simulink model "Powertrain_model_HEV_21a"  (R2021a)
settings: Solver=VariableStepAuto  StartTime=0.0  StopTime=tspan  RelTol=1e-3
values from neighbouring files (symbols this model uses):
  bsfc_idle_CE = 31.7e03    (= 31700)    [Sim_script.m]
  bsfc_idle_GE = 4.96e03    (= 4960)    [Sim_script.m]
  DR = 5.213    [Sim_script.m]
  drawn_pow_M = 464.6018    [Sim_script.m]
  Gensetdata = Gensetdata1    [Sim_script.m]
  motor_eff = motor_eff_PMSM    [Sim_script.m]
  Trans_In = 24.086    [Sim_script.m]
  tspan = 10800    [Sim_script.m]
  w_CE_idle = 400    [Sim_script.m]
undefined symbols (not defined in the file or in its folder): dailyloadl, eta_EM_map, MaxLimit, resT_hybrid_bollard, resT_hybrid_free, resT_hybrid_tow, T_EM_col, T_EM_max, w_EM_row
libraries: pid_lib x1
settings Model: Creator=user  LastModifiedBy=olsonsao
settings SolverCC: AlgebraicLoopSolver=TrustRegion

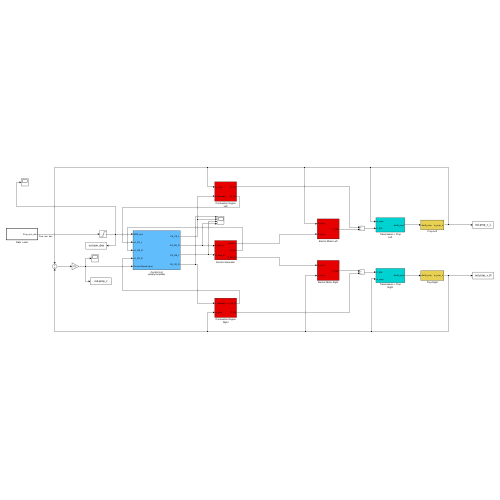
[thumbnail: Simulink's stored preview of the top-level diagram]
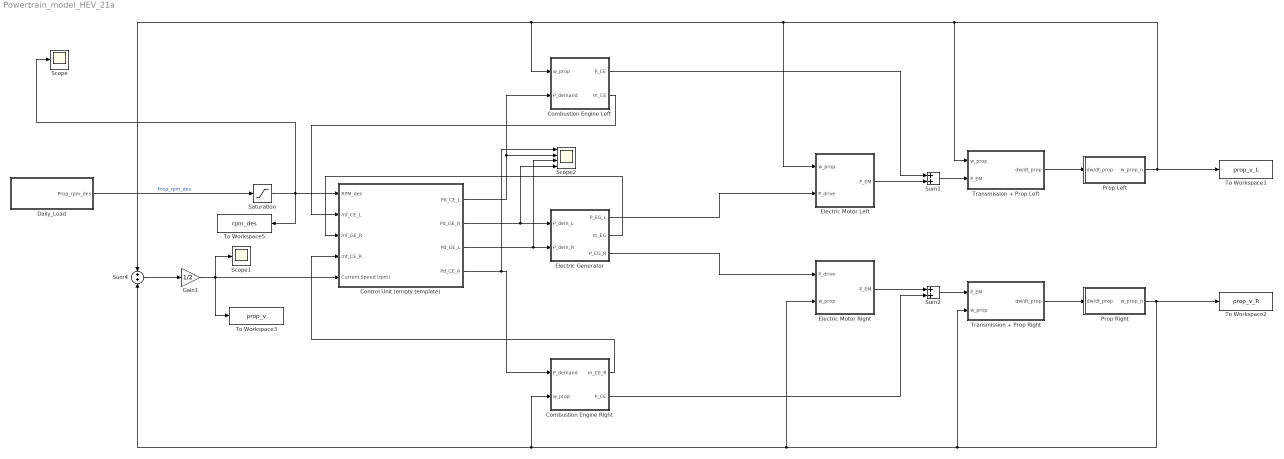
== system Powertrain_model_HEV_21a ==
  Combustion Engine Left : Subsystem  Tag=combustion engine
  Combustion Engine Right : Subsystem  Tag=combustion engine
  Control Unit (empty template) : Subsystem  Tag=control unit
  Daily_Load : Subsystem  TreatAsAtomicUnit=on
  "Electric Generator " : Subsystem
  Electric Motor Left : Subsystem
  Electric Motor Right : Subsystem
  Gain1 : Gain  Gain=1/2
  Prop Left : Subsystem
  Prop Right : Subsystem
  Saturation : Saturate  UpperLimit=inf  LowerLimit=w_CE_idle/DR
  Scope : Scope
  Scope1 : Scope
  Scope2 : Scope  NumInputPorts=4
  Sum1 : Sum
  Sum2 : Sum
  Sum4 : Sum  Inputs=+|+
  To Workspace1 : ToWorkspace  VariableName=prop_v_L  SampleTime=-1
      settings: Save2DSignal=2-D array (concatenate along first dimension)
  To Workspace2 : ToWorkspace  VariableName=prop_v_R  SampleTime=-1
      settings: Save2DSignal=2-D array (concatenate along first dimension)
  To Workspace3 : ToWorkspace  VariableName=prop_v  SampleTime=-1
      settings: Save2DSignal=2-D array (concatenate along first dimension)
  To Workspace5 : ToWorkspace  VariableName=rpm_des  SampleTime=-1
      settings: Save2DSignal=2-D array (concatenate along first dimension)
  Transmission + Prop Left : Subsystem
  Transmission + Prop Right : Subsystem
  wires:
  Transmission + Prop Left/1(dw/dt_prop) -> Prop Left/1(dw/dt_prop)
  Transmission + Prop Right/1(dw/dt_prop) -> Prop Right/1(dw/dt_prop)
  Prop Left/1(w_prop_n) -> Transmission + Prop Left/1(w_prop), Electric Motor Left/1(w_prop), Sum4/1, Combustion Engine Left/1(w_prop), To Workspace1/1
  Electric Motor Right/1(P_EM) -> Sum2/1
  Sum2/1 -> Transmission + Prop Right/1(P_EM)
  Combustion Engine Left/1(P_CE) -> Sum1/1
  Sum1/1 -> Transmission + Prop Left/2(P_EM)
  Electric Motor Left/1(P_EM) -> Sum1/2
  Combustion Engine Right/1(m_CE_R) -> Control Unit (empty template)/4(mf_CE_R)
  Combustion Engine Left/2(m_CE) -> Control Unit (empty template)/2(mf_CE_L)
  Control Unit (empty template)/4(Pd_CE_R) -> Scope2/1, Combustion Engine Right/1(P_demand)
  Control Unit (empty template)/1(Pd_CE_L) -> Combustion Engine Left/2(P_demand), Scope2/2
  "Electric Generator "/2(m_EG) -> Control Unit (empty template)/3(mf_GE_R)
  Combustion Engine Right/2(P_CE) -> Sum2/2
  Saturation/1 -> Scope/1, To Workspace5/1, Control Unit (empty template)/1(RPM_des)
  Control Unit (empty template)/2(Pd_GE_R) -> Scope2/4, "Electric Generator "/1(P_dem_L)
  Sum4/1 -> Gain1/1
  Daily_Load/1(Prop_rpm_des) -> Saturation/1  "Prop_rpm_des"
  Control Unit (empty template)/3(Pd_GE_L) -> Scope2/3, "Electric Generator "/2(P_dem_R)
  "Electric Generator "/1(P_EG_L) -> Electric Motor Left/2(P_drive)
  "Electric Generator "/3(P_EG_R) -> Electric Motor Right/1(P_drive)
  Prop Right/1(w_prop_n) -> Transmission + Prop Right/2(w_prop), Electric Motor Right/2(w_prop), Combustion Engine Right/2(w_prop), Sum4/2, To Workspace2/1
  Gain1/1 -> To Workspace3/1, Scope1/1, Control Unit (empty template)/5(Current Speed (rpm))

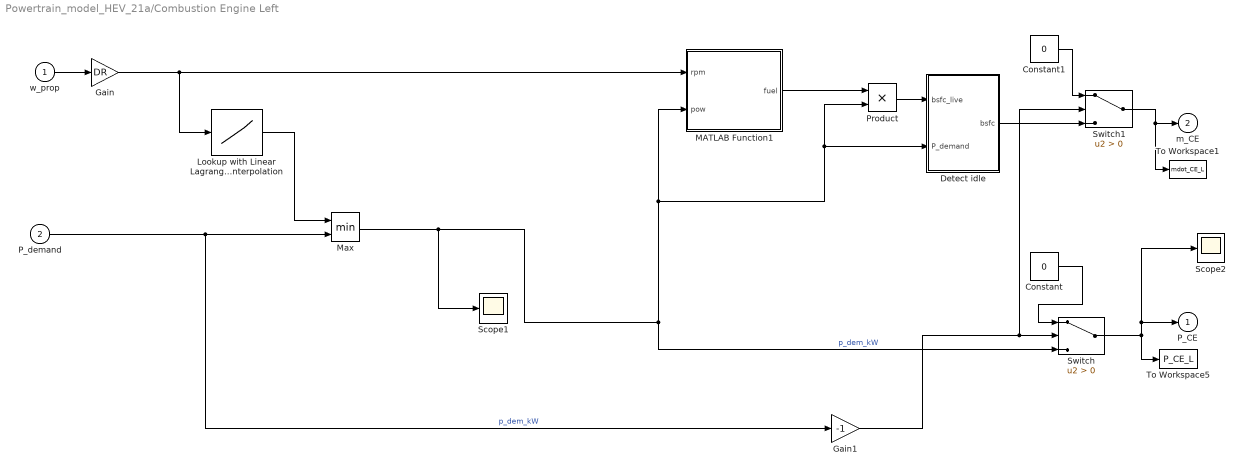
== system Powertrain_model_HEV_21a/Combustion Engine Left ==
  w_prop : Inport
  P_demand : Inport  Port=2
  Constant : Constant  Value=0
  Constant1 : Constant  Value=0
  Detect idle : Subsystem
  Gain : Gain  Gain=DR
  Gain1 : Gain  Gain=-1
  Lookup with Linear Lagrange Interpolation : Lookup_n-D  NumberOfTableDimensions=1  BreakpointsForDimension1=MaxLimit.('RPM')  Table=MaxLimit.('Pow_kW_')  InterpMethod=Linear Lagrange  InternalRulePriority=Speed  RndMeth=Simplest  InputSameDT=on
  MATLAB Function1 : MATLAB Function  TreatAsAtomicUnit=on
  Max : MinMax  Inputs=2
  Product : Product
  Scope1 : Scope
  Scope2 : Scope
  Switch : Switch  Criteria=u2 > Threshold
  Switch1 : Switch  Criteria=u2 > Threshold
  To Workspace1 : ToWorkspace  VariableName=mdot_CE_L  SampleTime=-1
      settings: Save2DSignal=2-D array (concatenate along first dimension)
  To Workspace5 : ToWorkspace  VariableName=P_CE_L  SampleTime=-1
      settings: Save2DSignal=2-D array (concatenate along first dimension)
  P_CE : Outport  InitialOutput=0
  m_CE : Outport  Port=2  InitialOutput=0
  wires:
  w_prop/1 -> Gain/1
  Lookup with Linear Lagrange Interpolation/1 -> Max/1
  MATLAB Function1/1(fuel) -> Product/1
  Gain/1 -> Lookup with Linear Lagrange Interpolation/1, MATLAB Function1/1(rpm)
  Max/1 -> Switch/3, Product/2, Detect idle/2(P_demand), MATLAB Function1/2(pow), Scope1/1  "p_dem_kW"
  P_demand/1 -> Gain1/1, Max/2  "p_dem_kW"
  Product/1 -> Detect idle/1(bsfc_live)
  Gain1/1 -> Switch1/2, Switch/2
  Constant/1 -> Switch/1
  Switch/1 -> Scope2/1, P_CE/1, To Workspace5/1
  Constant1/1 -> Switch1/1
  Detect idle/1(bsfc) -> Switch1/3
  Switch1/1 -> To Workspace1/1, m_CE/1

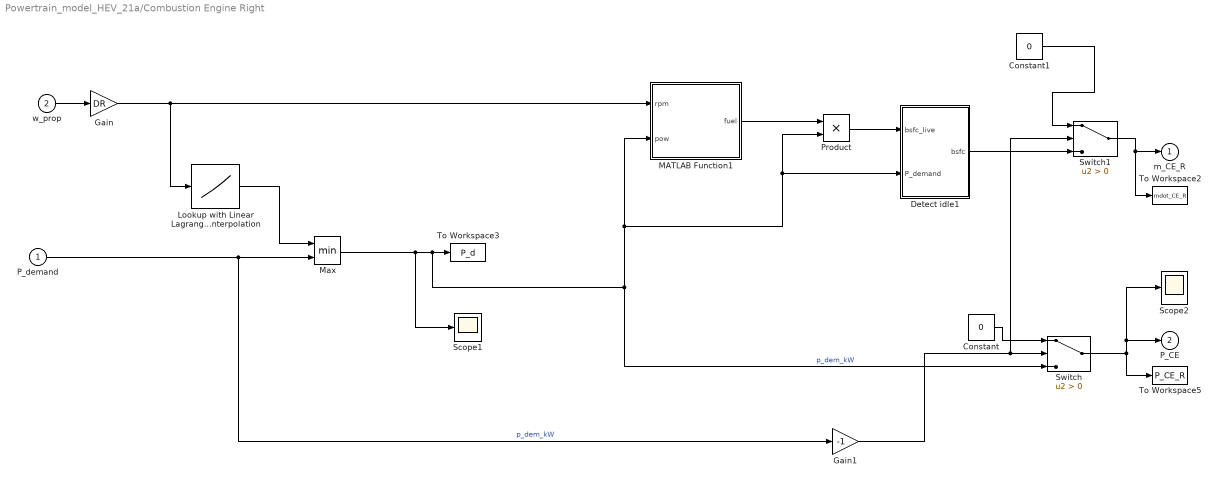
== system Powertrain_model_HEV_21a/Combustion Engine Right ==
  P_demand : Inport
  w_prop : Inport  Port=2
  Constant : Constant  Value=0
  Constant1 : Constant  Value=0
  Detect idle1 : Subsystem
  Gain : Gain  Gain=DR
  Gain1 : Gain  Gain=-1
  Lookup with Linear Lagrange Interpolation : Lookup_n-D  NumberOfTableDimensions=1  BreakpointsForDimension1=MaxLimit.('RPM')  Table=MaxLimit.('Pow_kW_')  InterpMethod=Linear Lagrange  InternalRulePriority=Speed  RndMeth=Simplest  InputSameDT=on
  MATLAB Function1 : MATLAB Function  TreatAsAtomicUnit=on
  Max : MinMax  Inputs=2
  Product : Product
  Scope1 : Scope
  Scope2 : Scope
  Switch : Switch  Criteria=u2 > Threshold
  Switch1 : Switch  Criteria=u2 > Threshold
  To Workspace2 : ToWorkspace  VariableName=mdot_CE_R  SampleTime=-1
      settings: Save2DSignal=2-D array (concatenate along first dimension)
  To Workspace3 : ToWorkspace  VariableName=P_d  SampleTime=-1
      settings: Save2DSignal=2-D array (concatenate along first dimension)
  To Workspace5 : ToWorkspace  VariableName=P_CE_R  SampleTime=-1
      settings: Save2DSignal=2-D array (concatenate along first dimension)
  m_CE_R : Outport  InitialOutput=0
  P_CE : Outport  Port=2  InitialOutput=0
  wires:
  w_prop/1 -> Gain/1
  Lookup with Linear Lagrange Interpolation/1 -> Max/1
  MATLAB Function1/1(fuel) -> Product/1
  Gain/1 -> Lookup with Linear Lagrange Interpolation/1, MATLAB Function1/1(rpm)
  Product/1 -> Detect idle1/1(bsfc_live)
  Max/1 -> Scope1/1, Switch/3, Detect idle1/2(P_demand), Product/2, MATLAB Function1/2(pow), To Workspace3/1  "p_dem_kW"
  Detect idle1/1(bsfc) -> Switch1/3
  Constant/1 -> Switch/1
  Gain1/1 -> Switch1/2, Switch/2
  P_demand/1 -> Gain1/1, Max/2  "p_dem_kW"
  Switch/1 -> Scope2/1, P_CE/1, To Workspace5/1
  Constant1/1 -> Switch1/1
  Switch1/1 -> To Workspace2/1, m_CE_R/1

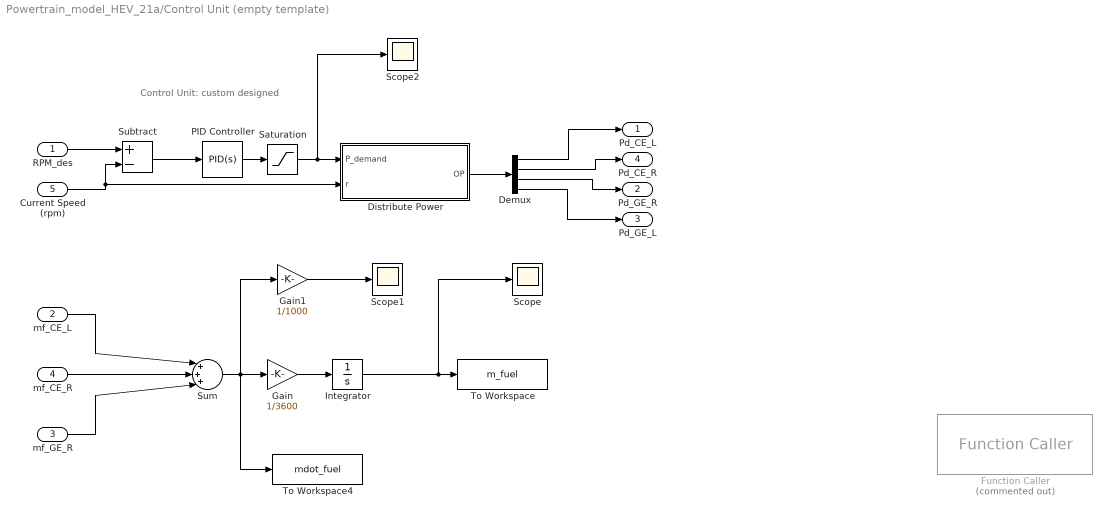
== system Powertrain_model_HEV_21a/Control Unit (empty template) ==
  note: Control Unit: custom designed
  RPM_des : Inport
  mf_CE_L : Inport  Port=2
  mf_GE_R : Inport  Port=3
  mf_CE_R : Inport  Port=4
  Current Speed (rpm) : Inport  Port=5
  Demux : Demux
  Distribute Power : MATLAB Function  TreatAsAtomicUnit=on
  Function Caller : FunctionCaller  Commented=on  FunctionPrototype=OP = power_distribute_func(power,rpm)  InputArgumentSpecifications=double(1),double(1)  OutputArgumentSpecifications=double([1,1,1,1])
  Gain : Gain  Gain=1/3600
  Gain1 : Gain  Gain=1/1000
  Integrator : Integrator
  PID Controller : pid_lib/PID Controller  Controller=PID  Form=Parallel  TimeDomain=Continuous-time  UseExternalTs=off  SampleTime=-1  IntegratorMethod=Forward Euler  FilterMethod=Forward Euler  ControllerParametersSource=internal  P=1.27731937948155  I=0.314602230470785  D=0.413734700213223  UseFilter=on  N=0.624884340967824  TunerSelectOption=Transfer Function Based (PID Tuner App)  InitialConditionSource=internal  InitialConditionForIntegrator=0  InitialConditionForFilter=0  DifferentiatorICPrevScaledInput=0  ExternalReset=none  TrackingMode=off  Kt=1  LimitOutput=on  SatLimitsSource=internal  UpperSaturationLimit=inf  LowerSaturationLimit=0  LinearizeAsGain=on  AntiWindupMode=none  Kb=1  POutMin=[]  POutMax=[]  IOutMin=[]  IOutMax=[]  DOutMin=[]  DOutMax=[]  NOutMin=[]  NOutMax=[]  SumOutMin=[]  SumOutMax=[]  SaturationOutMin=[]  SaturationOutMax=[]  PParamMin=[]  PParamMax=[]  IParamMin=[]  IParamMax=[]  DParamMin=[]  DParamMax=[]  NParamMin=[]  NParamMax=[]  KbParamMin=[]  KbParamMax=[]  KtParamMin=[]  KtParamMax=[]  KbOutMin=[]  KbOutMax=[]  KtOutMin=[]  KtOutMax=[]  IntegratorOutMin=[]  IntegratorOutMax=[]  FilterOutMin=[]  FilterOutMax=[]  SumI1OutMin=[]  SumI1OutMax=[]  SumI2OutMin=[]  SumI2OutMax=[]  SumI3OutMin=[]  SumI3OutMax=[]  SumI4OutMin=[]  SumI4OutMax=[]  SumDOutMin=[]  SumDOutMax=[]  DifferentiatorOutMin=[]  DifferentiatorOutMax=[]  FilterDiffOutCoefMin=[]  FilterDiffOutCoefMax=[]  ReciprocalOutMin=[]  ReciprocalOutMax=[]  SumDenOutMin=[]  SumDenOutMax=[]  SumNumOutMin=[]  SumNumOutMax=[]  DivideOutMin=[]  DivideOutMax=[]  UdiffTsProdOutMin=[]  UdiffTsProdOutMax=[]  NTsProdOutMin=[]  NTsProdOutMax=[]  UintegralTsProdOutMin=[]  UintegralTsProdOutMax=[]  UngainTsProdOutMin=[]  UngainTsProdOutMax=[]  IntegratorContinuousStateAttributes=''  IntegratorStateMustResolveToSignalObject=off  IntegratorRTWStateStorageClass=Auto  FilterContinuousStateAttributes=''  FilterStateMustResolveToSignalObject=off  FilterRTWStateStorageClass=Auto  ParallelPVariant=InternalParameters  IdealPVariant=Disabled  IVariant=InternalParameters  DVariant=InternalParameters  IntegratorVariant=Continuous  SatVariant=Enabled  AWVariant=Passthrough  PCopyVariant=Disabled  TRVariant=Disabled  FdbkBlocksVariant=Forward  IdealPFdbkVariant=Disabled  SatFdbkVariant=Disabled  DerivativeFilterVariant=ContFilter  NVariant=InternalParameters  NCopyVariant=Disabled  FilterICVariant=InternalICsFilter  IntegratorICVariant=InternalICs  ExternalResetVariant=Disabled  TRSumVariant=Passthrough  SumFdbkVariant=Disabled  SumVariant=Sum_PID  TsampFilterVariant=InternalTs  TsampNgainVariant=Passthrough  TsampIntegralVariant=Passthrough  ExternalSaturationOutDataTypeStr=Inherit: Same as second input
  Saturation : Saturate  UpperLimit=inf  LowerLimit=0
  Scope : Scope
  Scope1 : Scope
  Scope2 : Scope
  Subtract : Sum  Inputs=+-
  Sum : Sum  Inputs=|+++|
  To Workspace : ToWorkspace  VariableName=m_fuel  SampleTime=-1
      settings: Save2DSignal=2-D array (concatenate along first dimension)
  To Workspace4 : ToWorkspace  VariableName=mdot_fuel  SampleTime=-1
      settings: Save2DSignal=2-D array (concatenate along first dimension)
  Pd_CE_L : Outport  InitialOutput=0
  Pd_GE_R : Outport  Port=2  InitialOutput=0
  Pd_GE_L : Outport  Port=3  InitialOutput=0
  Pd_CE_R : Outport  Port=4  InitialOutput=0
  wires:
  Current Speed (rpm)/1 -> Distribute Power/2(r), Subtract/2
  RPM_des/1 -> Subtract/1
  Subtract/1 -> PID Controller/1
  mf_GE_R/1 -> Sum/3
  mf_CE_R/1 -> Sum/2
  PID Controller/1 -> Saturation/1
  Distribute Power/1(OP) -> Demux/1
  Demux/1 -> Pd_CE_L/1
  Demux/4 -> Pd_GE_L/1
  Demux/2 -> Pd_CE_R/1
  Demux/3 -> Pd_GE_R/1
  mf_CE_L/1 -> Sum/1
  Saturation/1 -> Scope2/1, Distribute Power/1(P_demand)
  Gain/1 -> Integrator/1
  Integrator/1 -> To Workspace/1, Scope/1
  Gain1/1 -> Scope1/1
  Sum/1 -> To Workspace4/1, Gain1/1, Gain/1

== system Powertrain_model_HEV_21a/Daily_Load ==
  1-D Lookup Table : Lookup_n-D  NumberOfTableDimensions=1  BreakpointsForDimension1=[1:10800]  Table=dailyloadl.('m_sec')  InternalRulePriority=Speed  RndMeth=Simplest  InputSameDT=on
  Clock : Clock
  To Workspace3 : ToWorkspace  VariableName=t  SampleTime=-1
      settings: Save2DSignal=2-D array (concatenate along first dimension)
  Prop_rpm_des : Outport
  wires:
  Clock/1 -> To Workspace3/1, 1-D Lookup Table/1
  1-D Lookup Table/1 -> Prop_rpm_des/1

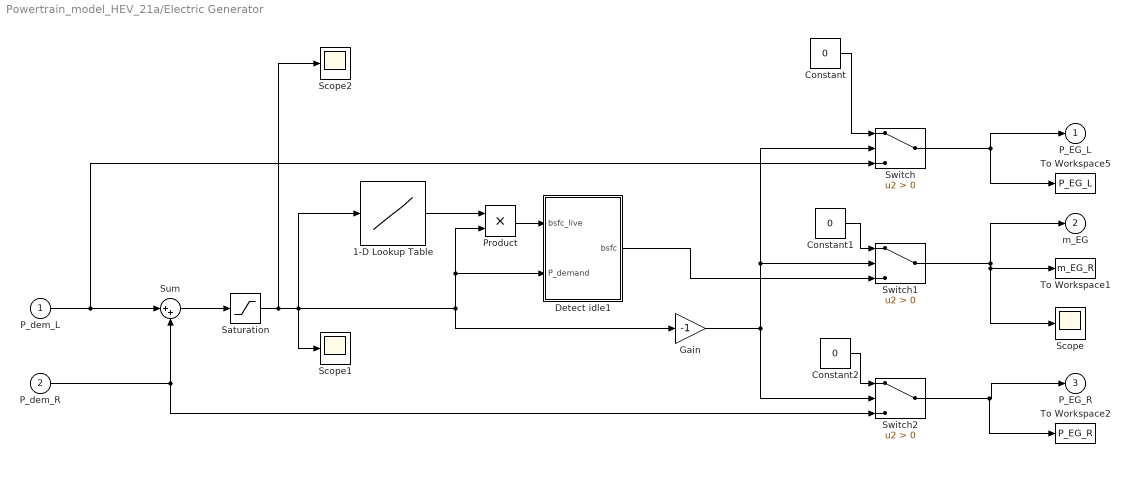
== system Powertrain_model_HEV_21a/Electric Generator  ==
  P_dem_L : Inport
  P_dem_R : Inport  Port=2
  1-D Lookup Table : Lookup_n-D  NumberOfTableDimensions=1  BreakpointsForDimension1=Gensetdata.('Power(kW)')  Table=Gensetdata.('Bsfc(g/kWh)')  InterpMethod=Cubic spline  ExtrapMethod=Cubic spline  InternalRulePriority=Speed  RndMeth=Simplest  InputSameDT=on
  Constant : Constant  Value=0
  Constant1 : Constant  Value=0
  Constant2 : Constant  Value=0
  Detect idle1 : Subsystem
  Gain : Gain  Gain=-1
  Product : Product
  Saturation : Saturate  UpperLimit=2500  LowerLimit=0
  Scope : Scope
  Scope1 : Scope
  Scope2 : Scope
  Sum : Sum  Inputs=|++
  Switch : Switch  Criteria=u2 > Threshold
  Switch1 : Switch  Criteria=u2 > Threshold
  Switch2 : Switch  Criteria=u2 > Threshold
  To Workspace1 : ToWorkspace  VariableName=m_EG_R  SampleTime=-1
      settings: Save2DSignal=2-D array (concatenate along first dimension)
  To Workspace2 : ToWorkspace  VariableName=P_EG_R  SampleTime=-1
      settings: Save2DSignal=2-D array (concatenate along first dimension)
  To Workspace5 : ToWorkspace  VariableName=P_EG_L  SampleTime=-1
      settings: Save2DSignal=2-D array (concatenate along first dimension)
  P_EG_L : Outport  InitialOutput=0
  m_EG : Outport  Port=2  InitialOutput=0
  P_EG_R : Outport  Port=3  InitialOutput=0
  wires:
  1-D Lookup Table/1 -> Product/1
  Saturation/1 -> Scope2/1, Scope1/1, Gain/1, Detect idle1/2(P_demand), Product/2, 1-D Lookup Table/1
  P_dem_L/1 -> Switch/3, Sum/1
  Sum/1 -> Saturation/1
  P_dem_R/1 -> Switch2/3, Sum/2
  Product/1 -> Detect idle1/1(bsfc_live)
  Constant/1 -> Switch/1
  Gain/1 -> Switch/2, Switch1/2, Switch2/2
  Constant1/1 -> Switch1/1
  Constant2/1 -> Switch2/1
  Detect idle1/1(bsfc) -> Switch1/3
  Switch/1 -> P_EG_L/1, To Workspace5/1
  Switch1/1 -> Scope/1, To Workspace1/1, m_EG/1
  Switch2/1 -> To Workspace2/1, P_EG_R/1

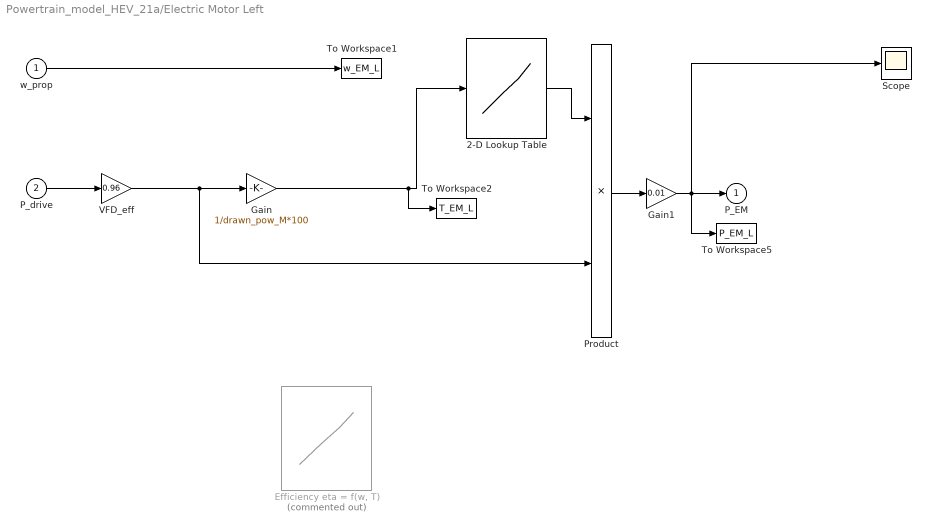
== system Powertrain_model_HEV_21a/Electric Motor Left ==
  w_prop : Inport
  P_drive : Inport  Port=2
  2-D Lookup Table : Lookup_n-D  NumberOfTableDimensions=1  BreakpointsForDimension1=motor_eff.('%power')  BreakpointsForDimension2=T_EM_col  Table=motor_eff.('eff')  InterpMethod=Cubic spline  ExtrapMethod=Cubic spline  InternalRulePriority=Speed  RndMeth=Simplest  InputSameDT=on
  "Efficiency eta = f(w, T)" : Lookup2D  Commented=on  RowIndex=w_EM_row  ColumnIndex=T_EM_col  Table=eta_EM_map
  Gain : Gain  Gain=1/drawn_pow_M*100
  Gain1 : Gain  Gain=0.01
  Product : Product  InputSameDT=on  RndMeth=Zero  SaturateOnIntegerOverflow=on  OutDataTypeStr=Inherit: Same as first input
  Scope : Scope
  To Workspace1 : ToWorkspace  VariableName=w_EM_L  SampleTime=-1
      settings: Save2DSignal=2-D array (concatenate along first dimension)
  To Workspace2 : ToWorkspace  VariableName=T_EM_L  SampleTime=-1
      settings: Save2DSignal=2-D array (concatenate along first dimension)
  To Workspace5 : ToWorkspace  VariableName=P_EM_L  SampleTime=-1
      settings: Save2DSignal=2-D array (concatenate along first dimension)
  VFD_eff : Gain  Gain=0.96
  P_EM : Outport  InitialOutput=0
  wires:
  Product/1 -> Gain1/1
  P_drive/1 -> VFD_eff/1
  2-D Lookup Table/1 -> Product/1
  w_prop/1 -> To Workspace1/1
  Gain/1 -> To Workspace2/1, 2-D Lookup Table/1
  VFD_eff/1 -> Gain/1, Product/2
  Gain1/1 -> Scope/1, To Workspace5/1, P_EM/1

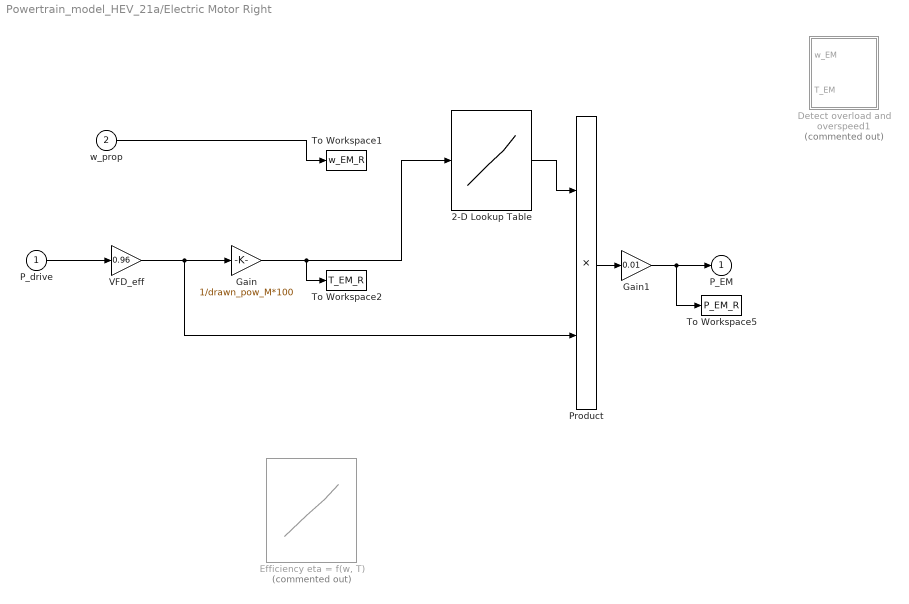
== system Powertrain_model_HEV_21a/Electric Motor Right ==
  P_drive : Inport
  w_prop : Inport  Port=2
  2-D Lookup Table : Lookup_n-D  NumberOfTableDimensions=1  BreakpointsForDimension1=motor_eff.('%power')  BreakpointsForDimension2=T_EM_col  Table=motor_eff.('eff')  InterpMethod=Cubic spline  ExtrapMethod=Cubic spline  InternalRulePriority=Speed  RndMeth=Simplest  InputSameDT=on
  Detect overload and overspeed1 : Subsystem  Commented=on
  "Efficiency eta = f(w, T)" : Lookup2D  Commented=on  RowIndex=w_EM_row  ColumnIndex=T_EM_col  Table=eta_EM_map
  Gain : Gain  Gain=1/drawn_pow_M*100
  Gain1 : Gain  Gain=0.01
  Product : Product  InputSameDT=on  RndMeth=Zero  SaturateOnIntegerOverflow=on  OutDataTypeStr=Inherit: Same as first input
  To Workspace1 : ToWorkspace  VariableName=w_EM_R  SampleTime=-1
      settings: Save2DSignal=2-D array (concatenate along first dimension)
  To Workspace2 : ToWorkspace  VariableName=T_EM_R  SampleTime=-1
      settings: Save2DSignal=2-D array (concatenate along first dimension)
  To Workspace5 : ToWorkspace  VariableName=P_EM_R  SampleTime=-1
      settings: Save2DSignal=2-D array (concatenate along first dimension)
  VFD_eff : Gain  Gain=0.96
  P_EM : Outport  InitialOutput=0
  wires:
  Product/1 -> Gain1/1
  P_drive/1 -> VFD_eff/1
  2-D Lookup Table/1 -> Product/1
  w_prop/1 -> To Workspace1/1
  Gain/1 -> To Workspace2/1, 2-D Lookup Table/1
  VFD_eff/1 -> Gain/1, Product/2
  Gain1/1 -> To Workspace5/1, P_EM/1

== system Powertrain_model_HEV_21a/Prop Left ==
  dw/dt_prop : Inport
  Gain : Gain  Gain=1/9.5493
  Integrator : Integrator  InitialCondition=w_CE_idle/DR  LowerSaturationLimit=1
  Saturation : Saturate  UpperLimit=inf  LowerLimit=0
  w_prop_n : Outport
  wires:
  dw/dt_prop/1 -> Integrator/1
  Integrator/1 -> Gain/1
  Saturation/1 -> w_prop_n/1
  Gain/1 -> Saturation/1

== system Powertrain_model_HEV_21a/Prop Right ==
  dw/dt_prop : Inport
  Gain : Gain  Gain=1/9.5493
  Integrator : Integrator  InitialCondition=w_CE_idle/DR  LowerSaturationLimit=1
  Saturation : Saturate  UpperLimit=inf  LowerLimit=0
  w_prop_n : Outport
  wires:
  dw/dt_prop/1 -> Integrator/1
  Integrator/1 -> Gain/1
  Saturation/1 -> w_prop_n/1
  Gain/1 -> Saturation/1

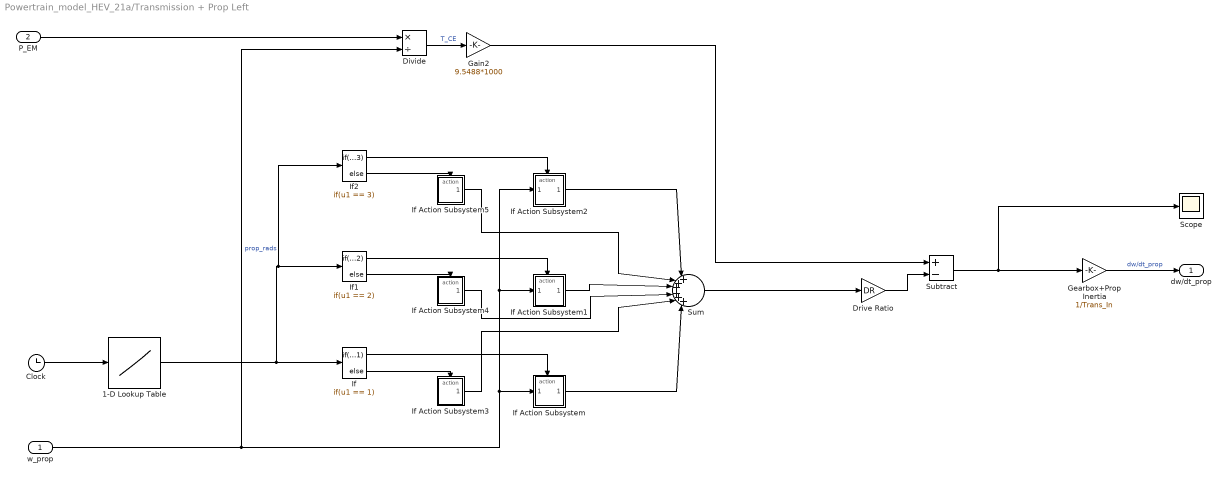
== system Powertrain_model_HEV_21a/Transmission + Prop Left ==
  w_prop : Inport
  P_EM : Inport  Port=2
  1-D Lookup Table : Lookup_n-D  NumberOfTableDimensions=1  BreakpointsForDimension1=[1:tspan]  Table=dailyloadl.('m_mode')  InternalRulePriority=Speed  RndMeth=Simplest  InputSameDT=on
  Clock : Clock
  Divide : Product  Inputs=*/
  Drive Ratio : Gain  Gain=DR
  Gain2 : Gain  Gain=9.5488*1000
  Gearbox+Prop Inertia : Gain  Gain=1/Trans_In
  If : If  IfExpression=u1 == 1
  If Action Subsystem : Subsystem  TreatAsAtomicUnit=on
  If Action Subsystem1 : Subsystem  TreatAsAtomicUnit=on
  If Action Subsystem2 : Subsystem  TreatAsAtomicUnit=on
  If Action Subsystem3 : Subsystem  TreatAsAtomicUnit=on
  If Action Subsystem4 : Subsystem  TreatAsAtomicUnit=on
  If Action Subsystem5 : Subsystem  TreatAsAtomicUnit=on
  If1 : If  IfExpression=u1 == 2
  If2 : If  IfExpression=u1 == 3
  Scope : Scope
  Subtract : Sum  Inputs=+-
  Sum : Sum  Inputs=|++++++|
  dw/dt_prop : Outport
  wires:
  P_EM/1 -> Divide/1
  Gearbox+Prop Inertia/1 -> dw/dt_prop/1  "dw/dt_prop"
  Subtract/1 -> Gearbox+Prop Inertia/1, Scope/1
  Divide/1 -> Gain2/1  "T_CE"
  Gain2/1 -> Subtract/1
  w_prop/1 -> If Action Subsystem2/1(w_prop), If Action Subsystem1/1(w_prop), If Action Subsystem/1(w_prop), Divide/2  "prop_rads"
  Drive Ratio/1 -> Subtract/2
  1-D Lookup Table/1 -> If2/1, If1/1, If/1
  Clock/1 -> 1-D Lookup Table/1
  If/1 -> If Action Subsystem/Action
  If/2 -> If Action Subsystem3/Action
  If1/1 -> If Action Subsystem1/Action
  If2/1 -> If Action Subsystem2/Action
  If2/2 -> If Action Subsystem5/Action
  If1/2 -> If Action Subsystem4/Action
  If Action Subsystem2/1(Out1) -> Sum/1
  If Action Subsystem5/1(Out1) -> Sum/2
  If Action Subsystem/1(Out1) -> Sum/6
  If Action Subsystem3/1(Out1) -> Sum/5
  If Action Subsystem1/1(Out1) -> Sum/3
  If Action Subsystem4/1(Out1) -> Sum/4
  Sum/1 -> Drive Ratio/1

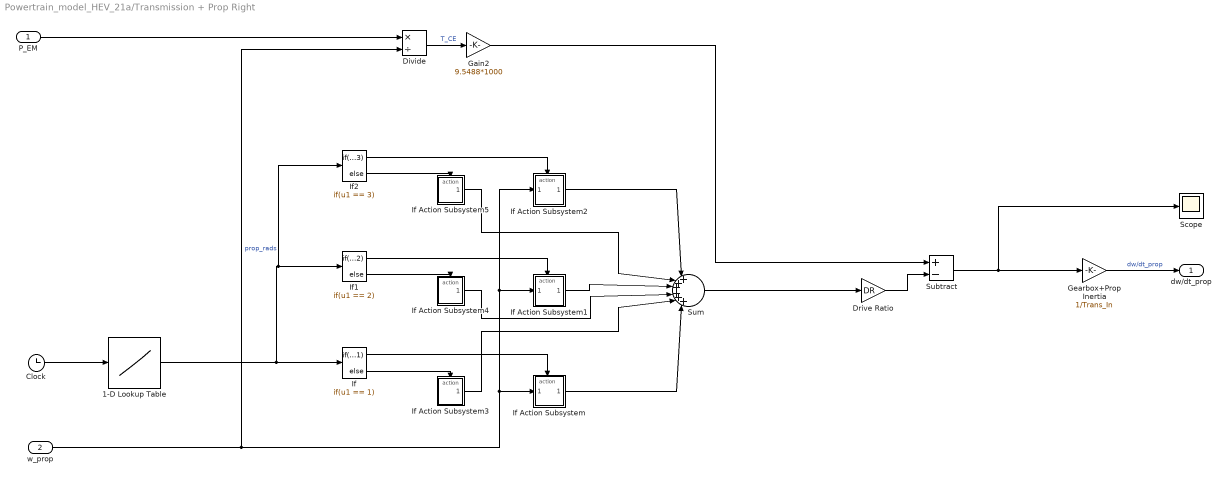
== system Powertrain_model_HEV_21a/Transmission + Prop Right ==
  P_EM : Inport
  w_prop : Inport  Port=2
  1-D Lookup Table : Lookup_n-D  NumberOfTableDimensions=1  BreakpointsForDimension1=[1:tspan]  Table=dailyloadl.('m_mode')  InternalRulePriority=Speed  RndMeth=Simplest  InputSameDT=on
  Clock : Clock
  Divide : Product  Inputs=*/
  Drive Ratio : Gain  Gain=DR
  Gain2 : Gain  Gain=9.5488*1000
  Gearbox+Prop Inertia : Gain  Gain=1/Trans_In
  If : If  IfExpression=u1 == 1
  If Action Subsystem : Subsystem  TreatAsAtomicUnit=on
  If Action Subsystem1 : Subsystem  TreatAsAtomicUnit=on
  If Action Subsystem2 : Subsystem  TreatAsAtomicUnit=on
  If Action Subsystem3 : Subsystem  TreatAsAtomicUnit=on
  If Action Subsystem4 : Subsystem  TreatAsAtomicUnit=on
  If Action Subsystem5 : Subsystem  TreatAsAtomicUnit=on
  If1 : If  IfExpression=u1 == 2
  If2 : If  IfExpression=u1 == 3
  Scope : Scope
  Subtract : Sum  Inputs=+-
  Sum : Sum  Inputs=|++++++|
  dw/dt_prop : Outport
  wires:
  P_EM/1 -> Divide/1
  Gearbox+Prop Inertia/1 -> dw/dt_prop/1  "dw/dt_prop"
  Subtract/1 -> Gearbox+Prop Inertia/1, Scope/1
  Divide/1 -> Gain2/1  "T_CE"
  Gain2/1 -> Subtract/1
  w_prop/1 -> If Action Subsystem2/1(w_prop), If Action Subsystem1/1(w_prop), If Action Subsystem/1(w_prop), Divide/2  "prop_rads"
  Drive Ratio/1 -> Subtract/2
  1-D Lookup Table/1 -> If2/1, If1/1, If/1
  Clock/1 -> 1-D Lookup Table/1
  If/1 -> If Action Subsystem/Action
  If/2 -> If Action Subsystem3/Action
  If1/1 -> If Action Subsystem1/Action
  If2/1 -> If Action Subsystem2/Action
  If2/2 -> If Action Subsystem5/Action
  If1/2 -> If Action Subsystem4/Action
  If Action Subsystem2/1(Out1) -> Sum/1
  If Action Subsystem5/1(Out1) -> Sum/2
  If Action Subsystem/1(Out1) -> Sum/6
  If Action Subsystem3/1(Out1) -> Sum/5
  If Action Subsystem1/1(Out1) -> Sum/3
  If Action Subsystem4/1(Out1) -> Sum/4
  Sum/1 -> Drive Ratio/1

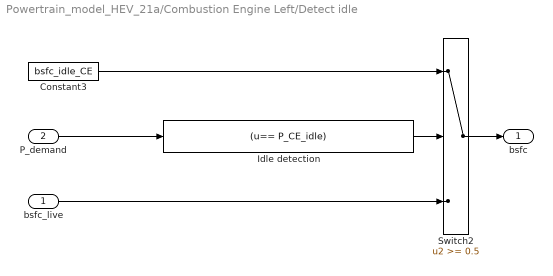
== system Powertrain_model_HEV_21a/Combustion Engine Left/Detect idle ==
  bsfc_live : Inport
  P_demand : Inport  Port=2
  Constant3 : Constant  Value=bsfc_idle_CE
  Idle detection : Fcn  Expr=(u== P_CE_idle)
  Switch2 : Switch  Threshold=0.5  SaturateOnIntegerOverflow=on  InputSameDT=on
  bsfc : Outport  InitialOutput=0
  wires:
  P_demand/1 -> Idle detection/1
  Idle detection/1 -> Switch2/2
  bsfc_live/1 -> Switch2/3
  Switch2/1 -> bsfc/1
  Constant3/1 -> Switch2/1

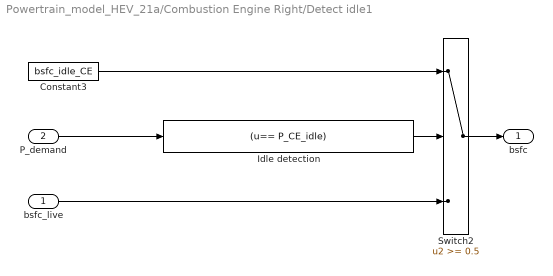
== system Powertrain_model_HEV_21a/Combustion Engine Right/Detect idle1 ==
  bsfc_live : Inport
  P_demand : Inport  Port=2
  Constant3 : Constant  Value=bsfc_idle_CE
  Idle detection : Fcn  Expr=(u== P_CE_idle)
  Switch2 : Switch  Threshold=0.5  SaturateOnIntegerOverflow=on  InputSameDT=on
  bsfc : Outport  InitialOutput=0
  wires:
  P_demand/1 -> Idle detection/1
  Idle detection/1 -> Switch2/2
  bsfc_live/1 -> Switch2/3
  Switch2/1 -> bsfc/1
  Constant3/1 -> Switch2/1

== system Powertrain_model_HEV_21a/Electric Generator /Detect idle1 ==
  bsfc_live : Inport
  P_demand : Inport  Port=2
  Constant3 : Constant  Value=bsfc_idle_GE
  Idle detection : Fcn  Expr=(u== P_CE_idle)
  Switch2 : Switch  Threshold=0.5  SaturateOnIntegerOverflow=on  InputSameDT=on
  bsfc : Outport  InitialOutput=0
  wires:
  P_demand/1 -> Idle detection/1
  Idle detection/1 -> Switch2/2
  bsfc_live/1 -> Switch2/3
  Switch2/1 -> bsfc/1
  Constant3/1 -> Switch2/1

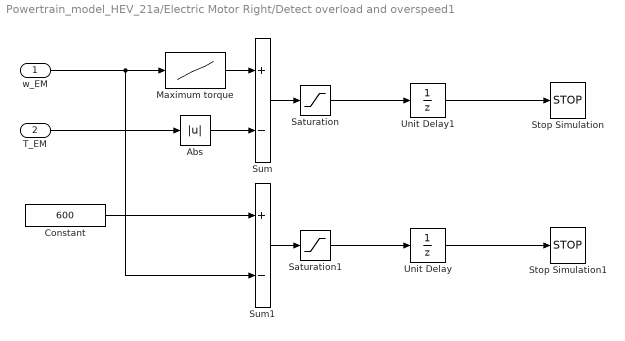
== system Powertrain_model_HEV_21a/Electric Motor Right/Detect overload and overspeed1 ==
  w_EM : Inport
  T_EM : Inport  Port=2
  Abs : Abs  SaturateOnIntegerOverflow=on
  Constant : Constant  Value=600
  Maximum torque : Lookup  InputValues=w_EM_row  Table=T_EM_max  SaturateOnIntegerOverflow=on
  Saturation : Saturate  UpperLimit=0  LowerLimit=-inf
  Saturation1 : Saturate  UpperLimit=0  LowerLimit=-inf
  Stop Simulation : Stop
  Stop Simulation1 : Stop
  Sum : Sum  Inputs=+-  InputSameDT=on  SaturateOnIntegerOverflow=on  OutDataTypeStr=Inherit: Same as first input
  Sum1 : Sum  Inputs=+-  InputSameDT=on  SaturateOnIntegerOverflow=on  OutDataTypeStr=Inherit: Same as first input
  Unit Delay : UnitDelay  SampleTime=-1  HasFrameUpgradeWarning=on
  Unit Delay1 : UnitDelay  SampleTime=-1  HasFrameUpgradeWarning=on
  wires:
  Saturation1/1 -> Unit Delay/1
  Sum1/1 -> Saturation1/1
  Constant/1 -> Sum1/1
  Saturation/1 -> Unit Delay1/1
  Abs/1 -> Sum/2
  Maximum torque/1 -> Sum/1
  T_EM/1 -> Abs/1
  w_EM/1 -> Sum1/2, Maximum torque/1
  Sum/1 -> Saturation/1
  Unit Delay/1 -> Stop Simulation1/1
  Unit Delay1/1 -> Stop Simulation/1

== system Powertrain_model_HEV_21a/Transmission + Prop Left/If Action Subsystem ==
  w_prop : Inport
  Action Port : ActionPort
  Gain : Gain  Gain=DR
  Lookup with Linear Point-slope Interpolation1 : Lookup_n-D  NumberOfTableDimensions=1  BreakpointsForDimension1=resT_hybrid_free.('rpm')  Table=resT_hybrid_free.('resT')  InternalRulePriority=Speed  RndMeth=Simplest  InputSameDT=on
  Out1 : Outport
  wires:
  Lookup with Linear Point-slope Interpolation1/1 -> Out1/1
  w_prop/1 -> Gain/1  "prop_rads"
  Gain/1 -> Lookup with Linear Point-slope Interpolation1/1

== system Powertrain_model_HEV_21a/Transmission + Prop Left/If Action Subsystem1 ==
  w_prop : Inport
  Action Port : ActionPort
  Gain1 : Gain  Gain=DR
  Lookup with Linear Point-slope Interpolation2 : Lookup_n-D  NumberOfTableDimensions=1  BreakpointsForDimension1=resT_hybrid_tow.('rpm')  Table=resT_hybrid_tow.('resT')  InternalRulePriority=Speed  RndMeth=Simplest  InputSameDT=on
  Out1 : Outport
  wires:
  Lookup with Linear Point-slope Interpolation2/1 -> Out1/1
  Gain1/1 -> Lookup with Linear Point-slope Interpolation2/1
  w_prop/1 -> Gain1/1  "prop_rads"

== system Powertrain_model_HEV_21a/Transmission + Prop Left/If Action Subsystem2 ==
  w_prop : Inport
  Action Port : ActionPort
  Gain3 : Gain  Gain=DR
  Lookup with Linear Point-slope Interpolation3 : Lookup_n-D  NumberOfTableDimensions=1  BreakpointsForDimension1=resT_hybrid_bollard.('rpm')  Table=resT_hybrid_bollard.('resT')  InternalRulePriority=Speed  RndMeth=Simplest  InputSameDT=on
  Out1 : Outport
  wires:
  Lookup with Linear Point-slope Interpolation3/1 -> Out1/1
  Gain3/1 -> Lookup with Linear Point-slope Interpolation3/1
  w_prop/1 -> Gain3/1  "prop_rads"

== system Powertrain_model_HEV_21a/Transmission + Prop Left/If Action Subsystem3 ==
  Action Port : ActionPort
  Constant : Constant  Value=0
  Out1 : Outport
  wires:
  Constant/1 -> Out1/1

== system Powertrain_model_HEV_21a/Transmission + Prop Left/If Action Subsystem4 ==
  Action Port : ActionPort
  Constant : Constant  Value=0
  Out1 : Outport
  wires:
  Constant/1 -> Out1/1

== system Powertrain_model_HEV_21a/Transmission + Prop Left/If Action Subsystem5 ==
  Action Port : ActionPort
  Constant : Constant  Value=0
  Out1 : Outport
  wires:
  Constant/1 -> Out1/1

== system Powertrain_model_HEV_21a/Transmission + Prop Right/If Action Subsystem ==
  w_prop : Inport
  Action Port : ActionPort
  Gain : Gain  Gain=DR
  Lookup with Linear Point-slope Interpolation1 : Lookup_n-D  NumberOfTableDimensions=1  BreakpointsForDimension1=resT_hybrid_free.('rpm')  Table=resT_hybrid_free.('resT')  InternalRulePriority=Speed  RndMeth=Simplest  InputSameDT=on
  Out1 : Outport
  wires:
  Lookup with Linear Point-slope Interpolation1/1 -> Out1/1
  w_prop/1 -> Gain/1  "prop_rads"
  Gain/1 -> Lookup with Linear Point-slope Interpolation1/1

== system Powertrain_model_HEV_21a/Transmission + Prop Right/If Action Subsystem1 ==
  w_prop : Inport
  Action Port : ActionPort
  Gain1 : Gain  Gain=DR
  Lookup with Linear Point-slope Interpolation2 : Lookup_n-D  NumberOfTableDimensions=1  BreakpointsForDimension1=resT_hybrid_tow.('rpm')  Table=resT_hybrid_tow.('resT')  InternalRulePriority=Speed  RndMeth=Simplest  InputSameDT=on
  Out1 : Outport
  wires:
  Lookup with Linear Point-slope Interpolation2/1 -> Out1/1
  Gain1/1 -> Lookup with Linear Point-slope Interpolation2/1
  w_prop/1 -> Gain1/1  "prop_rads"

== system Powertrain_model_HEV_21a/Transmission + Prop Right/If Action Subsystem2 ==
  w_prop : Inport
  Action Port : ActionPort
  Gain3 : Gain  Gain=DR
  Lookup with Linear Point-slope Interpolation3 : Lookup_n-D  NumberOfTableDimensions=1  BreakpointsForDimension1=resT_hybrid_bollard.('rpm')  Table=resT_hybrid_bollard.('resT')  InternalRulePriority=Speed  RndMeth=Simplest  InputSameDT=on
  Out1 : Outport
  wires:
  Lookup with Linear Point-slope Interpolation3/1 -> Out1/1
  Gain3/1 -> Lookup with Linear Point-slope Interpolation3/1
  w_prop/1 -> Gain3/1  "prop_rads"

== system Powertrain_model_HEV_21a/Transmission + Prop Right/If Action Subsystem3 ==
  Action Port : ActionPort
  Constant : Constant  Value=0
  Out1 : Outport
  wires:
  Constant/1 -> Out1/1

== system Powertrain_model_HEV_21a/Transmission + Prop Right/If Action Subsystem4 ==
  Action Port : ActionPort
  Constant : Constant  Value=0
  Out1 : Outport
  wires:
  Constant/1 -> Out1/1

== system Powertrain_model_HEV_21a/Transmission + Prop Right/If Action Subsystem5 ==
  Action Port : ActionPort
  Constant : Constant  Value=0
  Out1 : Outport
  wires:
  Constant/1 -> Out1/1

== matlab function Powertrain_model_HEV_21a/Control Unit (empty template)/Distribute Power ==
  data: P_demand input; OP output; r input
function OP = callmyfunc(P_demand, r)
    OP = power_distribute_func(P_demand,r);
end

== matlab function Powertrain_model_HEV_21a/Combustion Engine Right/MATLAB Function1 ==
  data: rpm input; fuel output; pow input
function fuel = bsfc_map(rpm,pow)

    fuel = fuel_con_map(rpm,pow);
end

== matlab function Powertrain_model_HEV_21a/Combustion Engine Left/MATLAB Function1 ==
  data: rpm input; fuel output; pow input
function fuel = bsfc_map(rpm,pow)

    fuel = fuel_con_map(rpm,pow);
end
